simulink model "FKKinematics_DEG"  (R2025b)
settings: Solver=VariableStepAuto  StartTime=0.0  StopTime=10.0  RelTol=1e-3
settings Model: Creator=ahmed  LastModifiedBy=ahmed

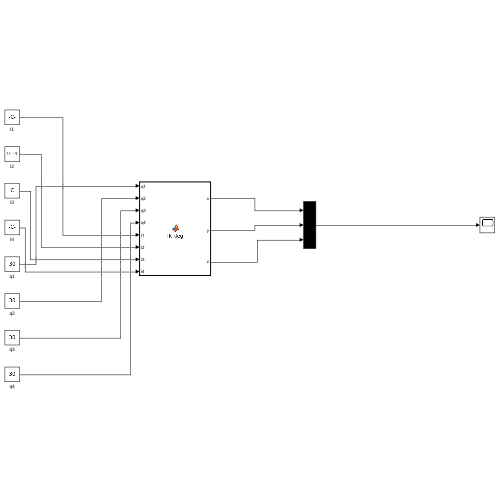
[thumbnail: Simulink's stored preview of the top-level diagram]
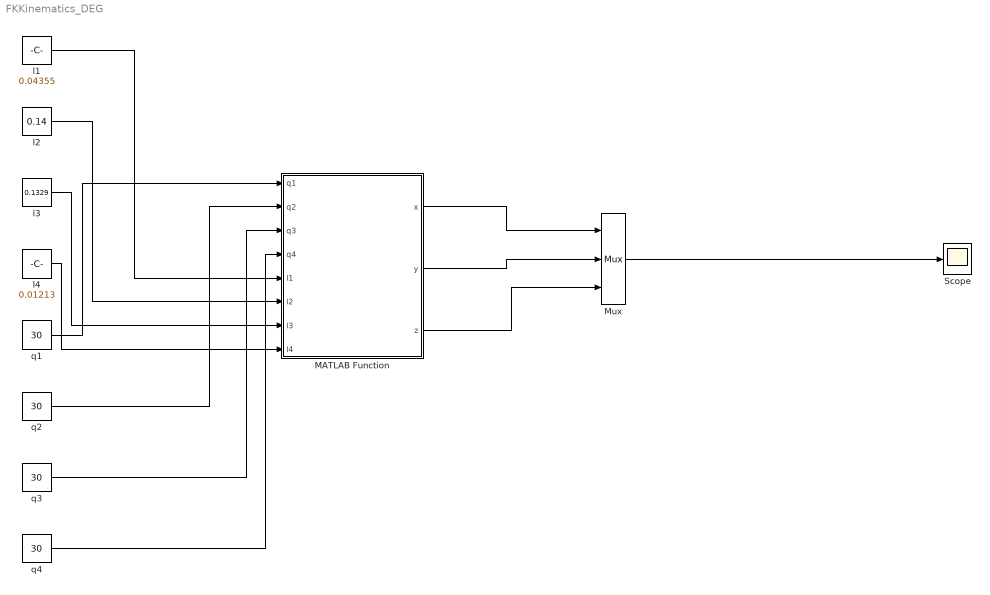
== system FKKinematics_DEG ==
  MATLAB Function : MATLAB Function  TreatAsAtomicUnit=on
  Mux : Mux  Inputs=3
  Scope : Scope
      settings: ActiveDisplayYMinimum=-0.10581018071593704  ActiveDisplayYMaximum=0.35419940305480041
  l1 : Constant  Value=0.04355
  l2 : Constant  Value=0.14
  l3 : Constant  Value=0.1329
  l4 : Constant  Value=0.01213
  q{1..4} (4 alike) : Constant  Value=30
  wires:
  l1/1 -> MATLAB Function/5(l1)
  l2/1 -> MATLAB Function/6(l2)
  l3/1 -> MATLAB Function/7(l3)
  l4/1 -> MATLAB Function/8(l4)
  q1/1 -> MATLAB Function/1(q1)
  q2/1 -> MATLAB Function/2(q2)
  q3/1 -> MATLAB Function/3(q3)
  q4/1 -> MATLAB Function/4(q4)
  Mux/1 -> Scope/1
  MATLAB Function/1(x) -> Mux/1
  MATLAB Function/2(y) -> Mux/2
  MATLAB Function/3(z) -> Mux/3

== matlab function FKKinematics_DEG/MATLAB Function ==
  data: x output; q1 input; y output; q2 input; q3 input; q4 input; l1 input; l2 input; l3 input; l4 input; z output
function [x,y,z] = fk_deg(q1,q2,q3,q4,l1,l2,l3,l4)
% Forward position from your exact matrices (DEGREES).
% Inputs: q1..q4 in degrees; l1..l4 in meters
% Outputs: x,y,z (meters)

x = l4*sin((q1*pi)/180) + l2*cos((q1*pi)/180)*cos((pi*(q2 + 90))/180) + l4*cos((q4*pi)/180)*(cos((q1*pi)/180)*cos((q3*pi)/180)*cos((pi*(q2 + 90))/180) + cos((q1*pi)/180)*sin((q3*pi)/180)*sin((pi*(q2 + 90))/180)) - l4*sin((q4*pi)/180)*(cos((q1*pi)/180)*cos((q3*pi)/180)*sin((pi*(q2 + 90))/180) - cos((q1*pi)/180)*sin((q3*pi)/180)*cos((pi*(q2 + 90))/180)) + l3*cos((q1*pi)/180)*cos((q3*pi)/180)*cos((pi*(q2 + 90))/180) + l3*cos((q1*pi)/180)*sin((q3*pi)/180)*sin((pi*(q2 + 90))/180);
y = l2*sin((q1*pi)/180)*cos((pi*(q2 + 90))/180) - l4*cos((q1*pi)/180) + l4*cos((q4*pi)/180)*(cos((q3*pi)/180)*sin((q1*pi)/180)*cos((pi*(q2 + 90))/180) + sin((q1*pi)/180)*sin((q3*pi)/180)*sin((pi*(q2 + 90))/180)) - l4*sin((q4*pi)/180)*(cos((q3*pi)/180)*sin((q1*pi)/180)*sin((pi*(q2 + 90))/180) - sin((q1*pi)/180)*sin((q3*pi)/180)*cos((pi*(q2 + 90))/180)) + l3*cos((q3*pi)/180)*sin((q1*pi)/180)*cos((pi*(q2 + 90))/180) + l3*sin((q1*pi)/180)*sin((q3*pi)/180)*sin((pi*(q2 + 90))/180);
z = l1 + l2*sin((pi*(q2 + 90))/180) + l3*cos((q3*pi)/180)*sin((pi*(q2 + 90))/180) - l3*sin((q3*pi)/180)*cos((pi*(q2 + 90))/180) + l4*cos((q4*pi)/180)*(cos((q3*pi)/180)*sin((pi*(q2 + 90))/180) - sin((q3*pi)/180)*cos((pi*(q2 + 90))/180)) + l4*sin((q4*pi)/180)*(cos((q3*pi)/180)*cos((pi*(q2 + 90))/180) + sin((q3*pi)/180)*sin((pi*(q2 + 90))/180));
